simulink model "beluga_vel_control_linear"  (R2016b)
settings: Solver=FixedStepAuto  StartTime=0.0  StopTime=10.0  FixedStep=0.001  RelTol=1e-3
values from neighbouring files (symbols this model uses):
  A = 1.06    [beluga_velocity_control_test.m]    (also in test_2.m = 0.0467438)
  desired_velocity = 0.5    [beluga_velocity_control_test.m]
  Kd = 0.3    [beluga_velocity_control_test.m]
  Ki = 3.77    [beluga_velocity_control_test.m]
  Kp = 20.2    [beluga_velocity_control_test.m]
  tau = 1.75    [beluga_velocity_control_test.m]
  tau_d = 0.09    [beluga_velocity_control_test.m]
libraries: simulink x1
settings Model: Creator=HMCLoaner  LastModifiedBy=HMCLoaner
settings OptimizationCC: LifeSpan=inf
settings DebuggingCC: SFExecutionAtInitializationDiag=none

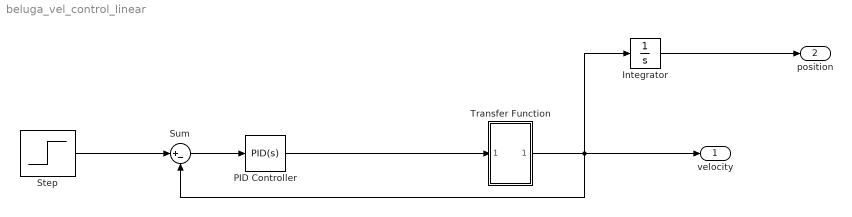
== system beluga_vel_control_linear ==
  Integrator : Integrator
  PID Controller : simulink/Continuous/PID Controller  Controller=PID  TimeDomain=Continuous-time  SampleTime=-1  IntegratorMethod=Forward Euler  FilterMethod=Forward Euler  Form=Parallel  UseFilter=on  ControllerParametersSource=internal  P=Kp  I=Ki  D=Kd  N=100  InitialConditionSource=internal  InitialConditionForIntegrator=0  InitialConditionForFilter=0  ExternalReset=none  LimitOutput=off  UpperSaturationLimit=inf  LowerSaturationLimit=-inf  LinearizeAsGain=on  AntiWindupMode=none  Kb=1  TrackingMode=off  Kt=1  PParamMin=[]  PParamMax=[]  IParamMin=[]  IParamMax=[]  DParamMin=[]  DParamMax=[]  NParamMin=[]  NParamMax=[]  KbParamMin=[]  KbParamMax=[]  KtParamMin=[]  KtParamMax=[]  POutMin=[]  POutMax=[]  IOutMin=[]  IOutMax=[]  DOutMin=[]  DOutMax=[]  NOutMin=[]  NOutMax=[]  KbOutMin=[]  KbOutMax=[]  KtOutMin=[]  KtOutMax=[]  IntegratorOutMin=[]  IntegratorOutMax=[]  FilterOutMin=[]  FilterOutMax=[]  SumOutMin=[]  SumOutMax=[]  SumI1OutMin=[]  SumI1OutMax=[]  SumI2OutMin=[]  SumI2OutMax=[]  SumI3OutMin=[]  SumI3OutMax=[]  SumDOutMin=[]  SumDOutMax=[]  SaturationOutMin=[]  SaturationOutMax=[]  IntegratorContinuousStateAttributes=''  IntegratorStateMustResolveToSignalObject=off  IntegratorRTWStateStorageClass=Auto  FilterContinuousStateAttributes=''  FilterStateMustResolveToSignalObject=off  FilterRTWStateStorageClass=Auto  DifferentiatorICPrevScaledInput=0  DifferentiatorOutMin=[]  DifferentiatorOutMax=[]
  Step : Step  Time=0  After=desired_velocity  SampleTime=0.1
  Sum : Sum  Inputs=|+-
  "Transfer Function " : Subsystem  Tag=Dynamic Model
  "velocity " : Outport
  "position " : Outport  Port=2
  wires:
  Sum/1 -> PID Controller/1
  "Transfer Function "/1(Out1) -> Integrator/1, Sum/2, "velocity "/1
  PID Controller/1 -> "Transfer Function "/1(In1)
  Step/1 -> Sum/1
  Integrator/1 -> "position "/1

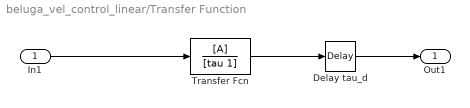
== system beluga_vel_control_linear/Transfer Function  ==
  In1 : Inport
  "Delay tau_d " : TransportDelay  DelayTime=tau_d
  Transfer Fcn : TransferFcn  Numerator=[A]  Denominator=[tau 1]
  Out1 : Outport
  wires:
  In1/1 -> Transfer Fcn/1
  Transfer Fcn/1 -> "Delay tau_d "/1
  "Delay tau_d "/1 -> Out1/1
